simulink model "chap11_2sim"  (Simulink 6.3)
settings: Solver=ode45  StartTime=0.0  StopTime=3  RelTol=1e-3
settings Model: LastModifiedBy=Administrator  ExtModeTrigMode=oneshot  ExtModeArmWhenConnect=off  StrictBusMsg=None
settings DataIOCC: LimitDataPoints=off
settings OptimizationCC: BlockReduction=off  BooleanDataType=off
settings DebuggingCC: SolverPrmCheckMsg=none
settings HardwareCC: TargetUnknown=on

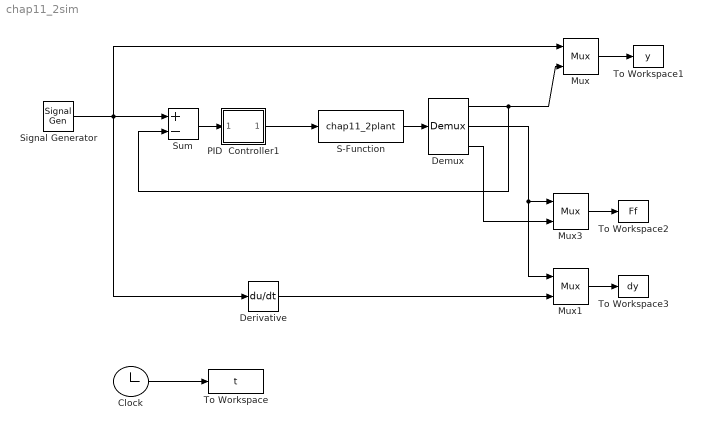
== system chap11_2sim ==
  Clock : Clock
      settings: Decimation=10
  Demux : Demux  Outputs=3
  Derivative : Derivative
  Mux : Mux  Inputs=2
  Mux1 : Mux  Inputs=2
  Mux3 : Mux  Inputs=2
  PID  Controller1 : Subsystem  mask(PID Controller){@1=200, @2=0, @3=40}
      mask prompts: @1 "Proportional:"; @2 "Integral"; @3 "Derivative:"
      mask help:
      | Enter expressions for proportional, integral, and derivative terms.
      | P+I/s+Ds
      mask init:
      | P=@1; I=@2; D=@3;
      mask Help: This block implements a PID controller where parameters are entered for the Proportional, Integral and Derivative terms. Unmask this block to see how it works. The derivative term is implemented using a true derivative block.
      mask Display: disp('PID')
  S-Function : S-Function  FunctionName=chap11_2plant
  Signal Generator : SignalGenerator  Amplitude=0.1
  Sum : Sum  Inputs=+-  SaturateOnIntegerOverflow=on  InputSameDT=on
  To Workspace : ToWorkspace  VariableName=t  SampleTime=-1  SaveFormat=Array
  To Workspace1 : ToWorkspace  VariableName=y  SampleTime=-1  SaveFormat=Array
  To Workspace2 : ToWorkspace  VariableName=Ff  SampleTime=-1  SaveFormat=Array
  To Workspace3 : ToWorkspace  VariableName=dy  SampleTime=-1  SaveFormat=Array
  wires:
  Sum/1 -> PID  Controller1/1(In_1)
  S-Function/1 -> Demux/1
  Mux/1 -> To Workspace1/1
  Demux/1 -> Mux/2, Sum/2
  PID  Controller1/1(Out_1) -> S-Function/1
  Demux/3 -> Mux3/2
  Demux/2 -> Mux1/1, Mux3/1
  Mux3/1 -> To Workspace2/1
  Mux1/1 -> To Workspace3/1
  Derivative/1 -> Mux1/2
  Signal Generator/1 -> Sum/1, Mux/1, Derivative/1
  Clock/1 -> To Workspace/1

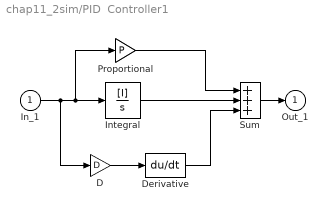
== system chap11_2sim/PID  Controller1 ==
  In_1 : Inport
  D : Gain  Gain=D  SaturateOnIntegerOverflow=on
  Derivative : Derivative
  Integral : TransferFcn  Numerator=[I]  Denominator=[1 0]
  Proportional : Gain  Gain=P  SaturateOnIntegerOverflow=on
  Sum : Sum  Inputs=+++  SaturateOnIntegerOverflow=on  InputSameDT=on
  Out_1 : Outport  InitialOutput=0
  wires:
  D/1 -> Derivative/1
  Sum/1 -> Out_1/1
  In_1/1 -> D/1, Proportional/1, Integral/1
  Derivative/1 -> Sum/3
  Integral/1 -> Sum/2
  Proportional/1 -> Sum/1
